simulink model "drone_position_estimate_continuous"  (R2020b)
settings: Solver=VariableStepAuto  StartTime=0.0  StopTime=30  RelTol=1e-3
values from neighbouring files (symbols this model uses):
  A = [zeros(3) eye(3)   zeros(3) ... (first row only)    [script_drone.m]
  B = [zeros(3) zeros(3) ... (first row only)    [script_drone.m]
  B_error = zeros(9,6)    [script_drone.m]
  C = [eye(3) zeros(3) zeros(3)]    [script_drone.m]
  D = [zeros(3) zeros(3)]    [script_drone.m]
  D_error = zeros(3,6)    [script_drone.m]
  F = A    [script_drone.m]
  G = [zeros(3) zeros(3) ... (first row only)    [script_drone.m]
  gps = zeros(3,1)    [script_drone.m]
  h = 0.1    [script_drone.m]
  H = C    [script_drone.m]
  h_plant = (1e-3)    (= 0.001)    [script_drone.m]
  L = lqed(F, G, H, Q, R, h)    [script_drone.m]
  Q = .1*eye(2*3)    [script_drone.m]
  R = .1*eye(3)    [script_drone.m]
  reference = [am;g]    [script_drone.m]
  sat_max = (10000)    (= 10000)    [script_drone.m]
  sat_min = -(10000)    (= -10000)    [script_drone.m]
  wind_final_value = 0    [script_drone.m]
  wind_initial_value = 0    [script_drone.m]
  wind_steptime = 5    [script_drone.m]
  x0 = zeros(n, 1)    [script_drone.m]
  x0_observer = zeros(n, 1)    [script_drone.m]
settings Model: Creator=lucas  LastModifiedBy=lucas

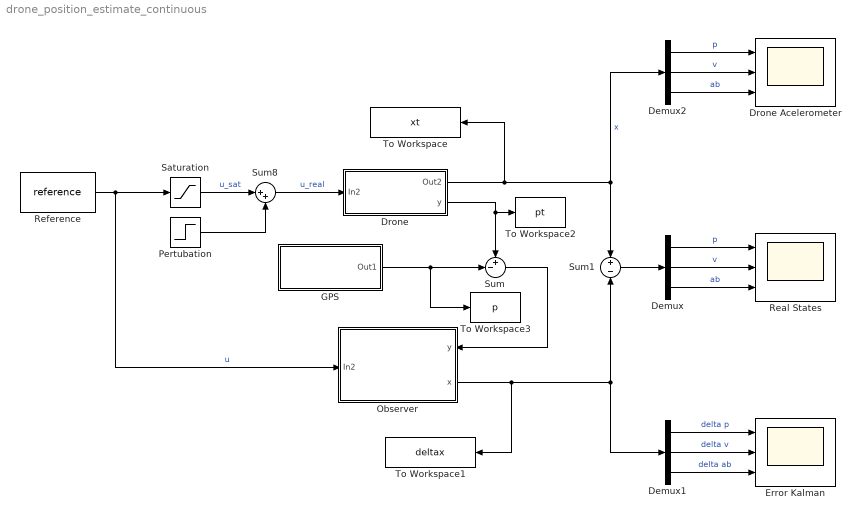
== system drone_position_estimate_continuous ==
  Demux : Demux  Outputs=3
  Demux1 : Demux  Outputs=3
  Demux2 : Demux  Outputs=3
  Drone : Subsystem
  Drone Acelerometer : Scope  NumInputPorts=3
  Error Kalman : Scope  NumInputPorts=3
  GPS : Subsystem
  Observer : Subsystem
      settings: PortSchema="{\"entries\":[{\"content\":{\"sides\":[{\"content\":{\"connectorIds\":[\"In1\"]},\"type\":\"ConnectorPlacement.EquallySpacedRectSide\",\"uuid\":\"b6dae28a-5485-44ef-84e6-2d14792229e7\"},{\"content\":{\"connectorIds\":[\"In2\",\"Out1\"],\"side\":\"RIGHT\"},\"type\":\"ConnectorPlacement.EquallySpacedRectSide\",\"uuid\":\"53a86c87-87d1-415f-9895-91b2b6ac7daf\"},{\"content\":{\"connectorIds\":[],\"side\":\"TOP\"},\"type\":\"ConnectorPlacement.EquallySpacedRectSide\",\"uuid\":\"c2916f3e-51bf-40f4-b6cd-eee6b60c38ec\"},{\"content\":{\"connectorIds\":[],\"side\":\"HIDDEN\"},\"type\":\"ConnectorPlacement.EquallySpacedRectSide\",\"uuid\":\"c85aafdf-e330-4d8d-a14a-206e12d7d836\"}]},\"type\":\"ConnectorPlacement.EquallySpacedConnector\",\"uuid\":\"08a8a426-31b9-42c2-8372-de3a4deaf2af\"}],\"packageUris\":[\"http://schema.mathworks.com/mf0/Connector/R2020b\"],\"version\":\"1.0\"}"
  Pertubation : Step  Time=wind_steptime  Before=wind_initial_value  After=wind_final_value  SampleTime=h_plant
  Real States : Scope  NumInputPorts=3
  Reference : Constant  Value=reference  SampleTime=h
  Saturation : Saturate  UpperLimit=sat_max  LowerLimit=sat_min
  Sum : Sum  Inputs=+-|
  Sum1 : Sum  Inputs=+|-
  Sum8 : Sum  Inputs=|++
  To Workspace : ToWorkspace  VariableName=xt  SaveFormat=Timeseries  SampleTime=-1
  To Workspace1 : ToWorkspace  VariableName=deltax  SaveFormat=Timeseries  SampleTime=-1
  To Workspace2 : ToWorkspace  VariableName=pt  SaveFormat=Timeseries  SampleTime=-1
  To Workspace3 : ToWorkspace  VariableName=p  SaveFormat=Timeseries  SampleTime=-1
  wires:
  Demux/3 -> Real States/3  "ab"
  Demux/1 -> Real States/1  "p"
  Demux/2 -> Real States/2  "v"
  Reference/1 -> Saturation/1, Observer/1(In2)  "u"
  Saturation/1 -> Sum8/1  "u_sat"
  Pertubation/1 -> Sum8/2
  Sum8/1 -> Drone/1(In2)  "u_real"
  Drone/2(y) -> To Workspace2/1, Sum/1
  Sum/1 -> Observer/2(y)
  Sum1/1 -> Demux/1
  Drone/1(Out2) -> To Workspace/1, Demux2/1, Sum1/1  "x"
  GPS/1(Out1) -> To Workspace3/1, Sum/2
  Observer/1(x) -> To Workspace1/1, Sum1/2, Demux1/1
  Demux1/1 -> Error Kalman/1  "delta p"
  Demux1/2 -> Error Kalman/2  "delta v"
  Demux1/3 -> Error Kalman/3  "delta ab"
  Demux2/3 -> Drone Acelerometer/3  "ab"
  Demux2/1 -> Drone Acelerometer/1  "p"
  Demux2/2 -> Drone Acelerometer/2  "v"

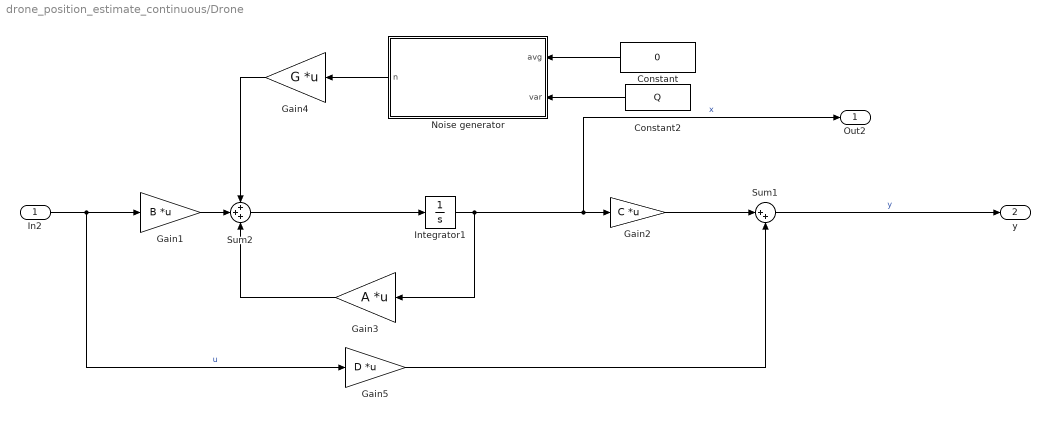
== system drone_position_estimate_continuous/Drone ==
  In2 : Inport
  Constant : Constant  Value=0  VectorParams1D=off
  Constant2 : Constant  Value=Q
  Gain1 : Gain  Gain=B  Multiplication=Matrix(K*u) (u vector)
  Gain2 : Gain  Gain=C  Multiplication=Matrix(K*u) (u vector)
  Gain3 : Gain  Gain=A  Multiplication=Matrix(K*u) (u vector)
  Gain4 : Gain  Gain=G  Multiplication=Matrix(K*u) (u vector)
  Gain5 : Gain  Gain=D  Multiplication=Matrix(K*u) (u vector)
  Integrator1 : Integrator  InitialCondition=x0
  Noise generator : MATLAB Function  TreatAsAtomicUnit=on
  Sum1 : Sum  Inputs=|++
  Sum2 : Sum  Inputs=+++
  Out2 : Outport
  y : Outport  Port=2
  wires:
  Sum2/1 -> Integrator1/1
  Gain2/1 -> Sum1/1
  Sum1/1 -> y/1  "y"
  In2/1 -> Gain5/1, Gain1/1  "u"
  Integrator1/1 -> Gain3/1, Out2/1, Gain2/1  "x"
  Gain1/1 -> Sum2/2
  Gain3/1 -> Sum2/3
  Noise generator/1(n) -> Gain4/1
  Gain4/1 -> Sum2/1
  Constant/1 -> Noise generator/1(avg)
  Constant2/1 -> Noise generator/2(var)
  Gain5/1 -> Sum1/2

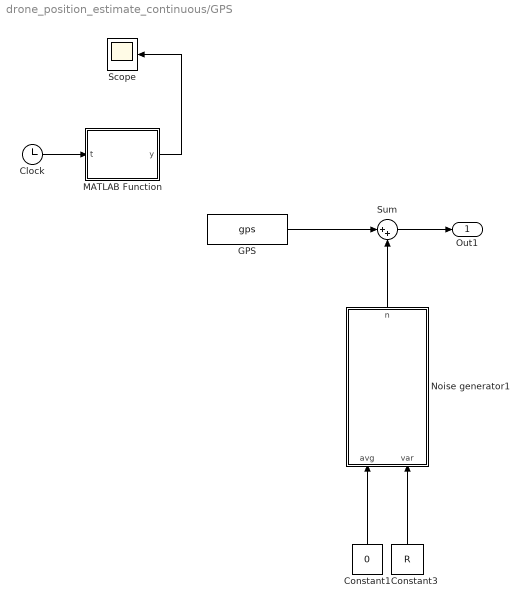
== system drone_position_estimate_continuous/GPS ==
  Clock : Clock
  Constant1 : Constant  Value=0
  Constant3 : Constant  Value=R
  GPS : Constant  Value=gps  VectorParams1D=off  SampleTime=h
  MATLAB Function : MATLAB Function  TreatAsAtomicUnit=on
  Noise generator1 : MATLAB Function  TreatAsAtomicUnit=on
  Scope : Scope
  Sum : Sum  Inputs=|++
  Out1 : Outport
  wires:
  Noise generator1/1(n) -> Sum/2
  Constant3/1 -> Noise generator1/2(var)
  Constant1/1 -> Noise generator1/1(avg)
  Sum/1 -> Out1/1
  Clock/1 -> MATLAB Function/1(t)
  MATLAB Function/1(y) -> Scope/1
  GPS/1 -> Sum/1

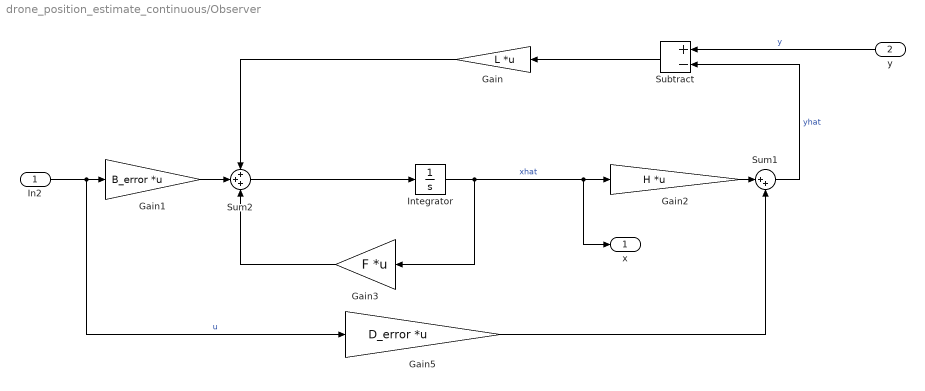
== system drone_position_estimate_continuous/Observer ==
  In2 : Inport
  y : Inport  Port=2
  Gain : Gain  Gain=L  Multiplication=Matrix(K*u) (u vector)
  Gain1 : Gain  Gain=B_error  Multiplication=Matrix(K*u) (u vector)
  Gain2 : Gain  Gain=H  Multiplication=Matrix(K*u) (u vector)
  Gain3 : Gain  Gain=F  Multiplication=Matrix(K*u) (u vector)
  Gain5 : Gain  Gain=D_error  Multiplication=Matrix(K*u) (u vector)
  Integrator : Integrator  InitialCondition=x0_observer
  Subtract : Sum  Inputs=+-
  Sum1 : Sum  Inputs=|++
  Sum2 : Sum  Inputs=+++
  x : Outport
  wires:
  Gain5/1 -> Sum1/2
  In2/1 -> Gain5/1, Gain1/1  "u"
  Sum2/1 -> Integrator/1
  Gain3/1 -> Sum2/3
  Integrator/1 -> Gain3/1, x/1, Gain2/1  "xhat"
  Gain1/1 -> Sum2/2
  Gain2/1 -> Sum1/1
  y/1 -> Subtract/1  "y"
  Sum1/1 -> Subtract/2  "yhat"
  Subtract/1 -> Gain/1
  Gain/1 -> Sum2/1

== matlab function drone_position_estimate_continuous/GPS/Noise generator1 ==
  data: avg input; n output; var input
function n = generate_gaussian_noise(avg, var)
n = avg + var*randn(length(var), 1);

== matlab function drone_position_estimate_continuous/Drone/Noise generator ==
  data: avg input; n output; var input
function n = generate_gaussian_noise(avg, var)
n = avg + var*randn(length(var), 1);

== matlab function drone_position_estimate_continuous/GPS/MATLAB Function ==
  data: t input; y output; x0 parameter
function y = fcn(t, x0)
    y = [0;0;(x0(3) + x0(6)*t -9.98*(t^2)/2)];
